simulink model "ex1b"  (R2015a)
settings: Solver=ode45  StartTime=0.0  StopTime=10.0  RelTol=1e-3
settings Model: Creator=ayush  LastModifiedBy=ayush

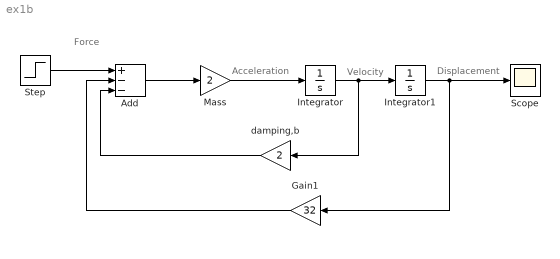
== system ex1b ==
  note: Force
  note: Displacement
  note: Velocity
  note: Acceleration
  Add : Sum  Inputs=+--
  Gain1 : Gain  Gain=32
  Integrator : Integrator
  Integrator1 : Integrator
  "Mass " : Gain  Gain=2
  Scope : Scope
  Step : Step  Time=0  After=10  SampleTime=0
  damping,b : Gain  Gain=2
  wires:
  Add/1 -> "Mass "/1
  "Mass "/1 -> Integrator/1
  Integrator/1 -> damping,b/1, Integrator1/1
  Integrator1/1 -> Gain1/1, Scope/1
  damping,b/1 -> Add/3
  Gain1/1 -> Add/2
  Step/1 -> Add/1
